simulink model "Exercise4"  (R2018b)
settings: Solver=VariableStepAuto  StartTime=0.0  StopTime=1  RelTol=1e-3
values from neighbouring files (symbols this model uses):
  fspeed = min(15*floor(time),255)    [Exercise3.m]
libraries: arduinolib x1
settings Model: Creator=tuxtorn  LastModifiedBy=tuxtorn

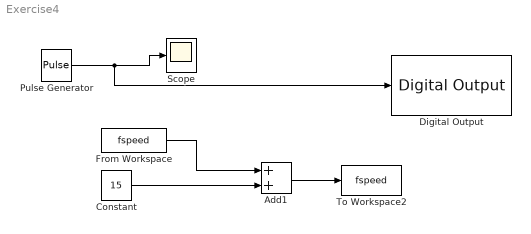
== system Exercise4 ==
  Add1 : Sum
  Constant : Constant  Value=15  SampleTime=1
  Digital Output : arduinolib/Digital Output  pinNumber=8  blockPlatform=arduino
  From Workspace : FromWorkspace  VariableName=fspeed
  Pulse Generator : DiscretePulseGenerator  PulseType=Time based  Period=0.001  PulseWidth=fspeed/255
  Scope : Scope
  To Workspace2 : ToWorkspace  VariableName=fspeed  SaveFormat=Timeseries  SampleTime=-1
  wires:
  Pulse Generator/1 -> Scope/1, Digital Output/1
  From Workspace/1 -> Add1/1
  Constant/1 -> Add1/2
  Add1/1 -> To Workspace2/1
